simulink model "LoopCounter"  (R2024b)
settings: Solver=VariableStepAuto  StartTime=0.0  StopTime=10.0  RelTol=1e-3
settings Model: Creator=ferbe  LastModifiedBy=ferbe
settings OptimizationCC: ReuseModelBlockBuffer=off
settings RTWCC: GPUComputeCapability=3.5

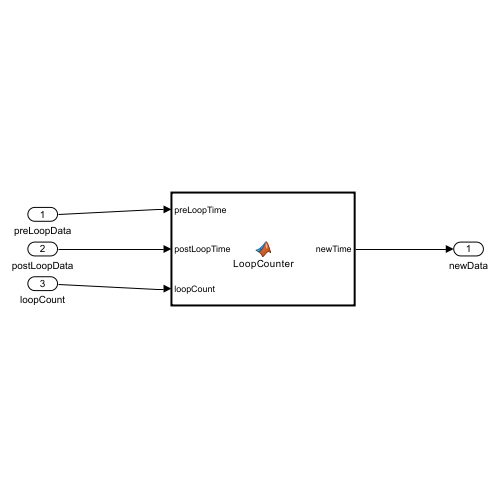
[thumbnail: Simulink's stored preview of the top-level diagram]
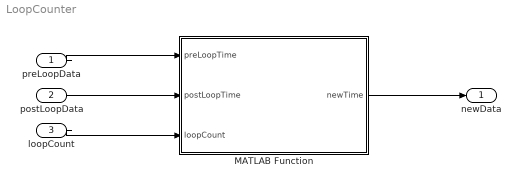
== system LoopCounter ==
  preLoopData : Inport
  postLoopData : Inport  Port=2
  loopCount : Inport  Port=3
  MATLAB Function : MATLAB Function  TreatAsAtomicUnit=on
  newData : Outport
  wires:
  MATLAB Function/1(newTime) -> newData/1
  preLoopData/1 -> MATLAB Function/1(preLoopTime)
  loopCount/1 -> MATLAB Function/3(loopCount)
  postLoopData/1 -> MATLAB Function/2(postLoopTime)

== matlab function LoopCounter/MATLAB Function ==
  data: preLoopTime input; newTime output; postLoopTime input; loopCount input
function newTime = LoopCounter(preLoopTime,postLoopTime,loopCount)
newTime = preLoopTime+loopCount*(postLoopTime-preLoopTime);
